simulink subsystem "bodyFM_to_thruster_forces"  (R2025b)
settings: Solver=VariableStepAuto  StartTime=0.0  StopTime=10.0  RelTol=1e-3
undefined symbols (not defined in the file or in its folder): invFT_wrench, invMT_wrench
settings Model: Creator=kjhaydon  LastModifiedBy=vulcangrip

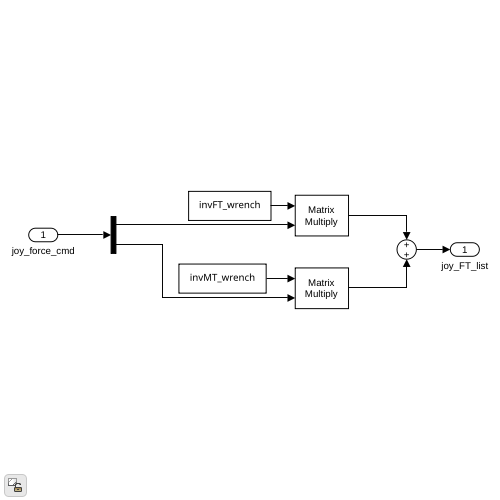
[thumbnail: Simulink's stored preview of the top-level diagram]
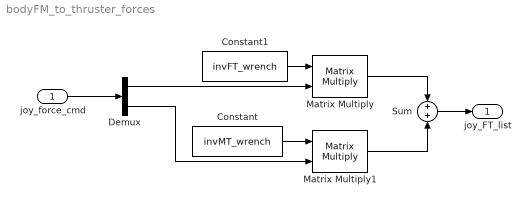
== system bodyFM_to_thruster_forces ==
  joy_force_cmd : Inport
  Constant : Constant  Value=invMT_wrench
  Constant1 : Constant  Value=invFT_wrench
  Demux : Demux  Outputs=2
  Matrix Multiply : Product  Multiplication=Matrix(*)
  Matrix Multiply1 : Product  Multiplication=Matrix(*)
  Sum : Sum
  joy_FT_list : Outport
  wires:
  joy_force_cmd/1 -> Demux/1
  Demux/1 -> Matrix Multiply/2
  Demux/2 -> Matrix Multiply1/2
  Constant/1 -> Matrix Multiply1/1
  Constant1/1 -> Matrix Multiply/1
  Matrix Multiply/1 -> Sum/1
  Matrix Multiply1/1 -> Sum/2
  Sum/1 -> joy_FT_list/1
